simulink model "unicycle_w_trailer"  (R2024b)
settings: Solver=VariableStepAuto  StartTime=0.0  StopTime=30  MaxStep=0.001  RelTol=1e-5
values from neighbouring files (symbols this model uses):
  K = 10    [init_params_unicycle.m]
  L = 10    [init_params_unicycle.m]
  q0 = [0; 10; pi/6; 0]    [init_params_unicycle.m]
  v = -2    [init_params_unicycle.m]
settings Model: Creator=Mathew  LastModifiedBy=rsimi
settings SolverCC: AlgebraicLoopSolver=TrustRegion
settings DebuggingCC: UnconnectedInputMsg=warning  UnconnectedOutputMsg=warning  UnconnectedLineMsg=warning
settings ModelReferenceCC: EnableRefExpFcnMdlSchedulingChecks=on
settings RTWCC: GPUComputeCapability=3.5  DLArmComputeVersion=19.05

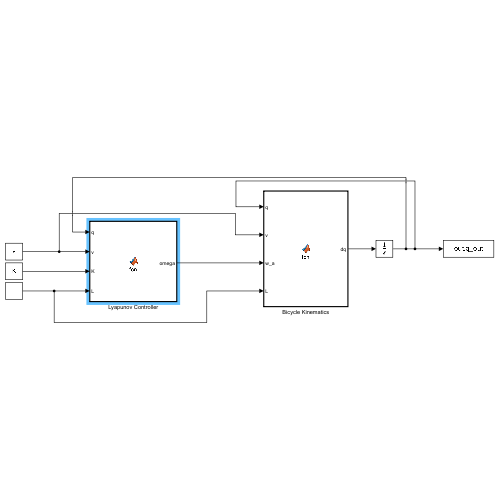
[thumbnail: Simulink's stored preview of the top-level diagram]
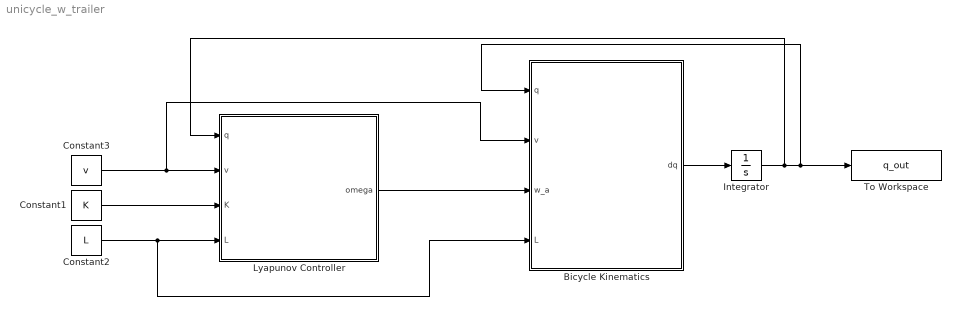
== system unicycle_w_trailer ==
  Bicycle Kinematics : MATLAB Function  TreatAsAtomicUnit=on
  Constant1 : Constant  Value=K
  Constant2 : Constant  Value=L
  Constant3 : Constant  Value=v
  Integrator : Integrator  InitialCondition=q0
  Lyapunov Controller : MATLAB Function  TreatAsAtomicUnit=on
  To Workspace : ToWorkspace  VariableName=q_out  SaveFormat=Timeseries  SampleTime=-1
  wires:
  Integrator/1 -> Lyapunov Controller/1(q), To Workspace/1, Bicycle Kinematics/1(q)
  Lyapunov Controller/1(omega) -> Bicycle Kinematics/3(w_a)
  Bicycle Kinematics/1(dq) -> Integrator/1
  Constant1/1 -> Lyapunov Controller/3(K)
  Constant2/1 -> Bicycle Kinematics/4(L), Lyapunov Controller/4(L)
  Constant3/1 -> Bicycle Kinematics/2(v), Lyapunov Controller/2(v)

== matlab function unicycle_w_trailer/Lyapunov Controller ==
  data: q input; omega output; v input; K input; L input
function omega  = fcn(q, v, K, L)

x = q(1);
y = q(2);
theta_a = q(3);
theta_p = q(4);

% control
omega = -y * v * sin(theta_a) / theta_a - K * theta_a;

== matlab function unicycle_w_trailer/Bicycle Kinematics ==
  data: q input; dq output; v input; w_a input; L input
function dq = fcn(q, v, w_a, L)

x_a = q(1); 
y_a = q(2); 
th_a = q(3);
th_p = q(4);

% Kinematics
dx_a = v * cos(th_a);
dy_a = v * sin(th_a);
dth_a = w_a;
dth_p = v * sin(th_a - th_p) / L;

dq = [dx_a ; dy_a ; dth_a; dth_p];
